simulink model "ddc_simulink_CRD"  (R2022b)
settings: Solver=VariableStepAuto  StartTime=0.0  StopTime=10.0  RelTol=1e-3
undefined symbols (not defined in the file): Fs, h, Ts
libraries: dspsrcs4 x1, dsphdlsigops2 x1
settings Model: Creator=caleb  LastModifiedBy=caleb

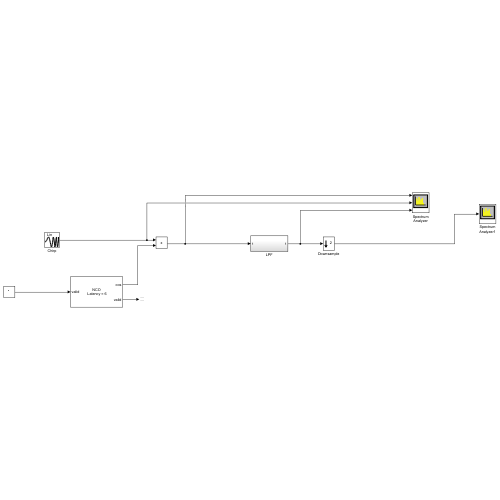
[thumbnail: Simulink's stored preview of the top-level diagram]
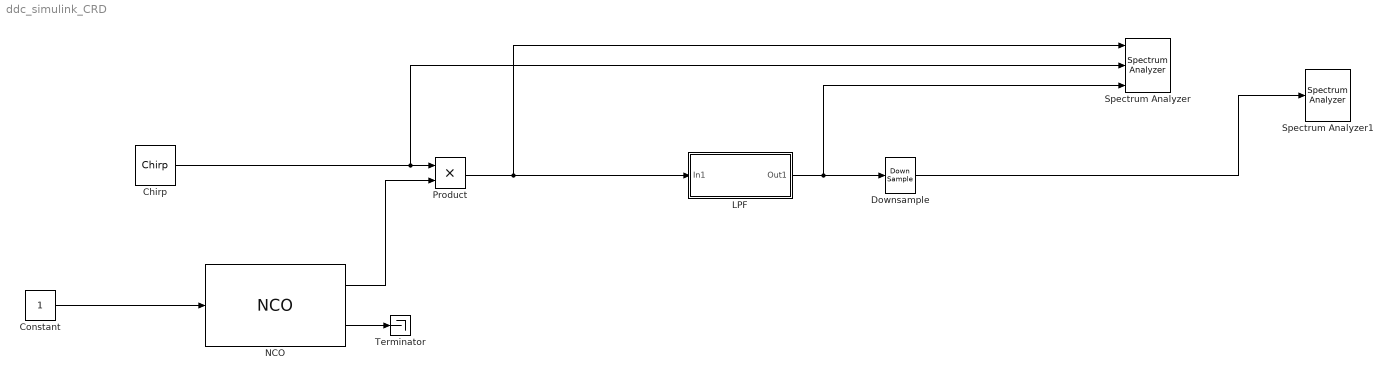
== system ddc_simulink_CRD ==
  Chirp : dspsrcs4/Chirp  sweep=Linear  mode=Unidirectional  f0=10e6  f1=20e6  t1=0.00001998  Tsweep=0.00001998  phase=0  Ts=1/Fs  spf=1  datatype=Double  OutputFrames=off
  Constant : Constant  OutDataTypeStr=boolean  SampleTime=Ts
  Downsample : DownSample  RateOptions=Allow multirate processing
  LPF : Subsystem
  NCO : dsphdlsigops2/NCO  PhaseIncrementSource=Property  PhaseIncrement=phIncr  PhaseOffsetSource=Property  PhaseOffset=phOff  DitherSource=Property  NumDitherBits=ditherBits  SamplesPerFrame=1  LUTCompress=off  ResetAction=off  Waveform=Cosine  PhasePort=off  SimulateUsing=Code generation  AccumulatorWL=N  PhaseQuantization=on  NumQuantizerAccumulatorBits=Q  OutputDataType=Binary point scaling  OutputWL=16  OutputFL=14
  Product : Product
  Spectrum Analyzer : SpectrumAnalyzer  NumInputPorts=3
  Spectrum Analyzer1 : SpectrumAnalyzer
  Terminator : Terminator
  wires:
  Constant/1 -> NCO/1
  NCO/1 -> Product/2
  Chirp/1 -> Spectrum Analyzer/2, Product/1
  Product/1 -> LPF/1(In1), Spectrum Analyzer/1
  LPF/1(Out1) -> Downsample/1, Spectrum Analyzer/3
  Downsample/1 -> Spectrum Analyzer1/1
  NCO/2 -> Terminator/1

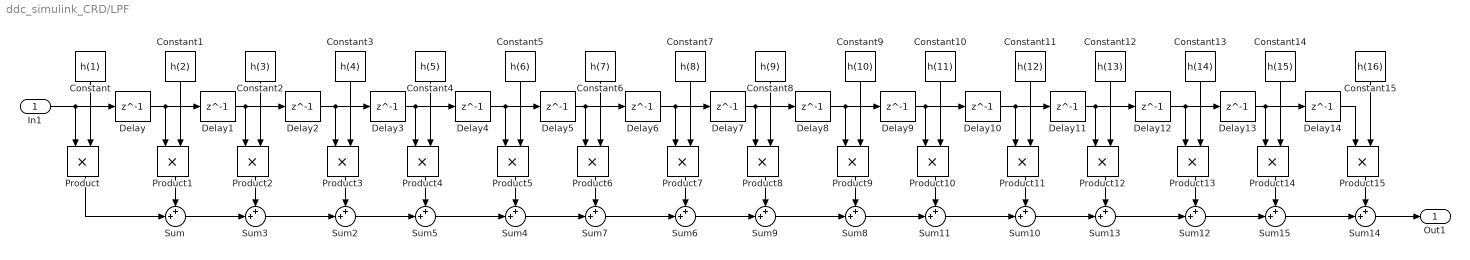
== system ddc_simulink_CRD/LPF ==
  In1 : Inport
  Constant : Constant  Value=h(1)
  Constant1 : Constant  Value=h(2)
  Constant10 : Constant  Value=h(11)
  Constant11 : Constant  Value=h(12)
  Constant12 : Constant  Value=h(13)
  Constant13 : Constant  Value=h(14)
  Constant14 : Constant  Value=h(15)
  Constant15 : Constant  Value=h(16)
  Constant2 : Constant  Value=h(3)
  Constant3 : Constant  Value=h(4)
  Constant4 : Constant  Value=h(5)
  Constant5 : Constant  Value=h(6)
  Constant6 : Constant  Value=h(7)
  Constant7 : Constant  Value=h(8)
  Constant8 : Constant  Value=h(9)
  Constant9 : Constant  Value=h(10)
  Delay{,1..14} (15 alike) : Delay  DelayLength=1  InitialCondition=0  UseCircularBuffer=on
  Product{,1..15} (16 alike) : Product
  Sum{,2..15} (15 alike) : Sum  Inputs=++|
  Out1 : Outport
  wires:
  In1/1 -> Delay/1, Product/1
  Delay/1 -> Product1/1, Delay1/1
  Constant/1 -> Product/2
  Constant1/1 -> Product1/2
  Product1/1 -> Sum/1
  Product/1 -> Sum/2
  Constant2/1 -> Product2/2
  Delay1/1 -> Delay2/1, Product2/1
  Product2/1 -> Sum3/1
  Delay2/1 -> Product3/1, Delay3/1
  Sum3/1 -> Sum2/2
  Constant3/1 -> Product3/2
  Product3/1 -> Sum2/1
  Constant4/1 -> Product4/2
  Delay3/1 -> Delay4/1, Product4/1
  Product4/1 -> Sum5/1
  Delay4/1 -> Product5/1, Delay5/1
  Sum5/1 -> Sum4/2
  Constant5/1 -> Product5/2
  Product5/1 -> Sum4/1
  Constant6/1 -> Product6/2
  Delay5/1 -> Delay6/1, Product6/1
  Product6/1 -> Sum7/1
  Delay6/1 -> Product7/1, Delay7/1
  Sum7/1 -> Sum6/2
  Constant7/1 -> Product7/2
  Product7/1 -> Sum6/1
  Constant8/1 -> Product8/2
  Delay7/1 -> Delay8/1, Product8/1
  Product8/1 -> Sum9/1
  Delay8/1 -> Product9/1, Delay9/1
  Sum9/1 -> Sum8/2
  Constant9/1 -> Product9/2
  Product9/1 -> Sum8/1
  Constant10/1 -> Product10/2
  Delay9/1 -> Delay10/1, Product10/1
  Product10/1 -> Sum11/1
  Delay10/1 -> Product11/1, Delay11/1
  Sum11/1 -> Sum10/2
  Constant11/1 -> Product11/2
  Product11/1 -> Sum10/1
  Constant12/1 -> Product12/2
  Delay11/1 -> Delay12/1, Product12/1
  Product12/1 -> Sum13/1
  Delay12/1 -> Product13/1, Delay13/1
  Sum13/1 -> Sum12/2
  Constant13/1 -> Product13/2
  Product13/1 -> Sum12/1
  Constant14/1 -> Product14/2
  Delay13/1 -> Delay14/1, Product14/1
  Product14/1 -> Sum15/1
  Delay14/1 -> Product15/1
  Sum15/1 -> Sum14/2
  Constant15/1 -> Product15/2
  Product15/1 -> Sum14/1
  Sum12/1 -> Sum15/2
  Sum10/1 -> Sum13/2
  Sum8/1 -> Sum11/2
  Sum6/1 -> Sum9/2
  Sum4/1 -> Sum7/2
  Sum2/1 -> Sum5/2
  Sum/1 -> Sum3/2
  Sum14/1 -> Out1/1
